simulink model "Hipertensooo"  (R2023a)
settings: Solver=ode15s  StartTime=0.0  StopTime=10  MaxStep=1e-3  RelTol=1e-3
libraries: slpidlib x1
settings Model: Creator=piqui  LastModifiedBy=jaelb
settings DataIOCC: ReturnWorkspaceOutputs=off  TimeSaveName=t
settings DebuggingCC: AlgebraicLoopMsg=none  ArtificialAlgebraicLoopMsg=none  MaxConsecutiveZCsMsg=none  ModelReferenceExtraNoncontSigs=none  OperatingPointInterfaceChecksumMismatchMsg=none

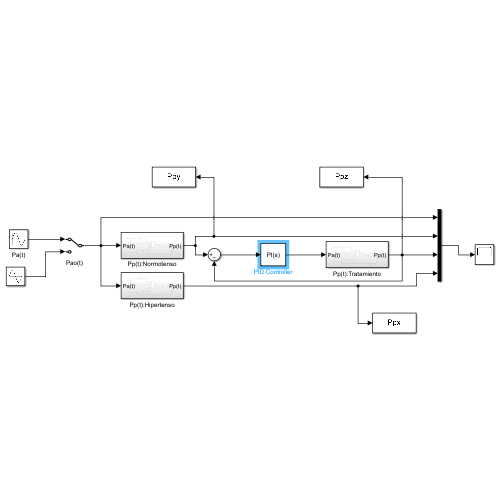
[thumbnail: Simulink's stored preview of the top-level diagram]
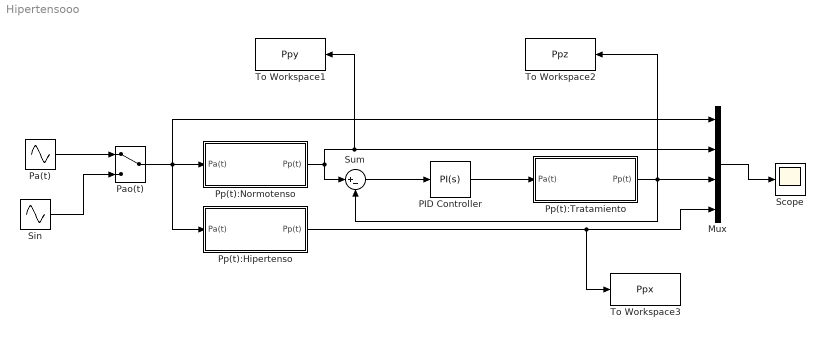
== system Hipertensooo ==
  Mux : Mux
  PID Controller : slpidlib/PID Controller  Controller=PI  Form=Parallel  TimeDomain=Continuous-time  UseExternalTs=off  SampleTime=-1  IntegratorMethod=Forward Euler  FilterMethod=Forward Euler  ControllerParametersSource=internal  P=0.00206448364843538  I=10333.3333  UseKiTs=off  D=0  N=100  UseFilter=on  TunerSelectOption=Transfer Function Based (PID Tuner App)  InitialConditionSource=internal  InitialConditionForIntegrator=0  InitialConditionForFilter=0  DifferentiatorICPrevScaledInput=0  ExternalReset=none  TrackingMode=off  Kt=1  LimitOutput=off  SatLimitsSource=internal  UpperSaturationLimit=inf  LowerSaturationLimit=-inf  LinearizeAsGain=on  AntiWindupMode=none  Kb=1  LimitIntegrator=off  UpperIntegratorSaturationLimit=inf  LowerIntegratorSaturationLimit=-inf  POutMin=[]  POutMax=[]  IOutMin=[]  IOutMax=[]  DOutMin=[]  DOutMax=[]  NOutMin=[]  NOutMax=[]  SumOutMin=[]  SumOutMax=[]  SaturationOutMin=[]  SaturationOutMax=[]  PParamMin=[]  PParamMax=[]  IParamMin=[]  IParamMax=[]  DParamMin=[]  DParamMax=[]  NParamMin=[]  NParamMax=[]  KbParamMin=[]  KbParamMax=[]  KtParamMin=[]  KtParamMax=[]  KbOutMin=[]  KbOutMax=[]  KtOutMin=[]  KtOutMax=[]  IntegratorOutMin=[]  IntegratorOutMax=[]  FilterOutMin=[]  FilterOutMax=[]  SumI1OutMin=[]  SumI1OutMax=[]  SumI2OutMin=[]  SumI2OutMax=[]  SumI3OutMin=[]  SumI3OutMax=[]  SumI4OutMin=[]  SumI4OutMax=[]  SumDOutMin=[]  SumDOutMax=[]  DifferentiatorOutMin=[]  DifferentiatorOutMax=[]  FilterDiffOutCoefMin=[]  FilterDiffOutCoefMax=[]  ReciprocalOutMin=[]  ReciprocalOutMax=[]  SumDenOutMin=[]  SumDenOutMax=[]  SumNumOutMin=[]  SumNumOutMax=[]  DivideOutMin=[]  DivideOutMax=[]  UdiffTsProdOutMin=[]  UdiffTsProdOutMax=[]  NTsProdOutMin=[]  NTsProdOutMax=[]  UintegralTsProdOutMin=[]  UintegralTsProdOutMax=[]  UngainTsProdOutMin=[]  UngainTsProdOutMax=[]  ClampingZeroOutDataTypeStr=Inherit: Inherit via back propagation  ClampingZeroOutMin=[]  ClampingZeroOutMax=[]  FilterDenConstantOutDataTypeStr=Inherit: Inherit via back propagation  FilterDenConstantOutMin=[]  FilterDenConstantOutMax=[]  PCopyOutDataTypeStr=Inherit: Inherit via back propagation  PCopyOutMin=[]  PCopyOutMax=[]  NCopyOutDataTypeStr=Inherit: Inherit via back propagation  NCopyOutMin=[]  NCopyOutMax=[]  IntegratorContinuousStateAttributes=''  IntegratorStateMustResolveToSignalObject=off  IntegratorRTWStateStorageClass=Auto  FilterContinuousStateAttributes=''  FilterStateMustResolveToSignalObject=off  FilterRTWStateStorageClass=Auto  ParallelPVariant=InternalParameters  IdealPVariant=Disabled  IVariant=InternalParameters  DVariant=Disabled  IntegratorVariant=Continuous  SatVariant=Disabled  AWVariant=Passthrough  PCopyVariant=Disabled  TRVariant=Disabled  FdbkBlocksVariant=Forward  IdealPFdbkVariant=Disabled  SatFdbkVariant=Disabled  DerivativeFilterVariant=Disabled  NVariant=Disabled  NCopyVariant=Disabled_SignalSpec  FilterICVariant=Disabled  IntegratorICVariant=InternalICs  ExternalResetVariant=Disabled  TRSumVariant=Passthrough  SumFdbkVariant=Disabled  SumVariant=Sum_PI  TsampFilterVariant=InternalTs  TsampNgainVariant=Passthrough  TsampIntegralVariant=Disabled_SignalSpec  ExternalSaturationOutDataTypeStr=Inherit: Same as second input
  Pa(t) : Sin  Bias=0.8  Frequency=(2*pi)*(95/60)
  Pao(t) : ManualSwitch
  Pp(t):Hipertenso : Subsystem
  Pp(t):Normotenso : Subsystem
  Pp(t):Tratamiento : Subsystem
  Scope : Scope
  Sin : Sin  Amplitude=1.5  Frequency=pi/2  SampleTime=0
  Sum : Sum  Inputs=|+-
  To Workspace1 : ToWorkspace  VariableName=Ppy  SampleTime=-1
  To Workspace2 : ToWorkspace  VariableName=Ppz  SampleTime=-1
  To Workspace3 : ToWorkspace  VariableName=Ppx  SampleTime=-1
  wires:
  Sum/1 -> PID Controller/1
  Pp(t):Normotenso/1(Pp(t)) -> Sum/1, To Workspace1/1, Mux/2
  Mux/1 -> Scope/1
  Pp(t):Hipertenso/1(Pp(t)) -> To Workspace3/1, Mux/4
  Pao(t)/1 -> Pp(t):Hipertenso/1(Pa(t)), Mux/1, Pp(t):Normotenso/1(Pa(t))
  Pa(t)/1 -> Pao(t)/1
  Sin/1 -> Pao(t)/2
  PID Controller/1 -> Pp(t):Tratamiento/1(Pa(t))
  Pp(t):Tratamiento/1(Pp(t)) -> To Workspace2/1, Sum/2, Mux/3

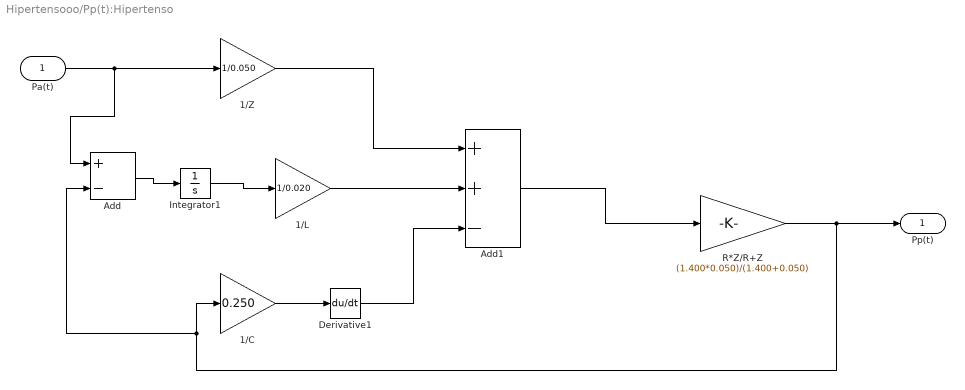
== system Hipertensooo/Pp(t):Hipertenso ==
  Pa(t) : Inport
  1/C : Gain  Gain=0.250
  1/L : Gain  Gain=1/0.020
  1/Z : Gain  Gain=1/0.050
  Add : Sum  Inputs=+-
  Add1 : Sum  Inputs=++-
  Derivative1 : Derivative
  Integrator1 : Integrator
  R*Z/R+Z : Gain  Gain=(1.400*0.050)/(1.400+0.050)
  Pp(t) : Outport
  wires:
  1/C/1 -> Derivative1/1
  Pa(t)/1 -> Add/1, 1/Z/1
  Add1/1 -> R*Z/R+Z/1
  1/Z/1 -> Add1/1
  Derivative1/1 -> Add1/3
  R*Z/R+Z/1 -> Add/2, 1/C/1, Pp(t)/1
  Add/1 -> Integrator1/1
  Integrator1/1 -> 1/L/1
  1/L/1 -> Add1/2

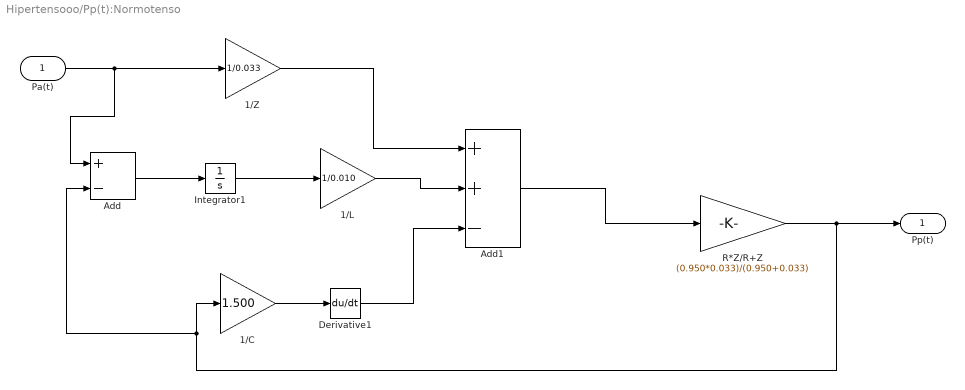
== system Hipertensooo/Pp(t):Normotenso ==
  Pa(t) : Inport
  1/C : Gain  Gain=1.500
  1/L : Gain  Gain=1/0.010
  1/Z : Gain  Gain=1/0.033
  Add : Sum  Inputs=+-
  Add1 : Sum  Inputs=++-
  Derivative1 : Derivative
  Integrator1 : Integrator
  R*Z/R+Z : Gain  Gain=(0.950*0.033)/(0.950+0.033)
  Pp(t) : Outport
  wires:
  1/C/1 -> Derivative1/1
  Pa(t)/1 -> Add/1, 1/Z/1
  Add1/1 -> R*Z/R+Z/1
  1/Z/1 -> Add1/1
  Derivative1/1 -> Add1/3
  R*Z/R+Z/1 -> Add/2, 1/C/1, Pp(t)/1
  Add/1 -> Integrator1/1
  Integrator1/1 -> 1/L/1
  1/L/1 -> Add1/2

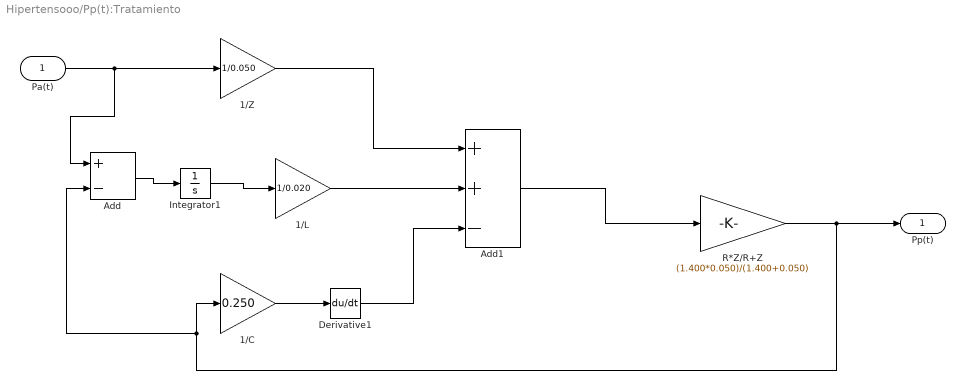
== system Hipertensooo/Pp(t):Tratamiento ==
  Pa(t) : Inport
  1/C : Gain  Gain=0.250
  1/L : Gain  Gain=1/0.020
  1/Z : Gain  Gain=1/0.050
  Add : Sum  Inputs=+-
  Add1 : Sum  Inputs=++-
  Derivative1 : Derivative
  Integrator1 : Integrator
  R*Z/R+Z : Gain  Gain=(1.400*0.050)/(1.400+0.050)
  Pp(t) : Outport
  wires:
  Derivative1/1 -> Add1/3
  1/Z/1 -> Add1/1
  Add1/1 -> R*Z/R+Z/1
  Pa(t)/1 -> Add/1, 1/Z/1
  Integrator1/1 -> 1/L/1
  1/L/1 -> Add1/2
  Add/1 -> Integrator1/1
  R*Z/R+Z/1 -> Add/2, 1/C/1, Pp(t)/1
  1/C/1 -> Derivative1/1
